simulink model "model_PD"  (R2016b)
settings: Solver=VariableStepAuto  StartTime=0.0  StopTime=30  FixedStep=Ts  RelTol=1e-3  EnableMultiTasking=on
values from neighbouring files (symbols this model uses):
  C = [eye(3),zeros(3,9);zeros(3,6),eye(3),zeros(3,3);zeros(3,9),eye(3)]    [model_script_Cascade.m]    (also in model_script_LQR_LQI.m; model_script_PD.m)
  D_height = .6117    (= 0.6117)    [model_script_Cascade.m]    (also in model_script_PD.m)
  D_pitch = .2256    (= 0.2256)    [model_script_Cascade.m]    (also in model_script_PD.m)
  D_roll = 0.1522    [model_script_Cascade.m]    (also in model_script_PD.m)
  D_yaw = .0367    (= 0.0367)    [model_script_Cascade.m]    (also in model_script_PD.m)
  g = 9.81    [model_script_Cascade.m]    (also in model_script_LQR_LQI.m; model_script_PD.m)
  I = diag([Ixx;Iyy;Izz])    [model_script_Cascade.m]    (also in model_script_LQR_LQI.m; model_script_PD.m)
  i0 = [tauphi;tautheta;taupsi;T]    [model_script_Cascade.m]    (also in model_script_LQR_LQI.m; model_script_PD.m)
  M = 0.487    [model_script_Cascade.m]    (also in model_script_LQR_LQI.m; model_script_PD.m)
  mean_att = zeros(3,1)    [model_script_Cascade.m]    (also in model_script_LQR_LQI.m; model_script_PD.m)
  mean_av = zeros(3,1)    [model_script_Cascade.m]    (also in model_script_LQR_LQI.m; model_script_PD.m)
  mean_pos = zeros(3,1)    [model_script_Cascade.m]    (also in model_script_LQR_LQI.m; model_script_PD.m)
  P_height = .3843    (= 0.3843)    [model_script_Cascade.m]    (also in model_script_PD.m)
  P_pitch = 1.9491    [model_script_Cascade.m]    (also in model_script_PD.m)
  P_roll = 1.5117    [model_script_Cascade.m]    (also in model_script_PD.m)
  P_yaw = .1152    (= 0.1152)    [model_script_Cascade.m]    (also in model_script_PD.m)
  propDistance = 0.125    [model_script_Cascade.m]    (also in model_script_LQR_LQI.m; model_script_PD.m)
  Q = diag([1e-5,1e-5,1e-5,1e-7,1e-7,1e-4,ones(1,2)*2e-7,6e-7,ones(1,3)*1e-7])    [model_script_Cascade.m]    (also in model_script_LQR_LQI.m; model_script_PD.m)
  R = diag(var)    [model_script_Cascade.m]    (also in model_script_LQR_LQI.m; model_script_PD.m)
  T_att = 1/200    (= 0.005)    [model_script_Cascade.m]    (also in model_script_LQR_LQI.m; model_script_PD.m)
  T_xy = 1/10    (= 0.1)    [model_script_Cascade.m]    (also in model_script_LQR_LQI.m; model_script_PD.m)
  T_yaw = 1/100    (= 0.01)    [model_script_Cascade.m]    (also in model_script_LQR_LQI.m; model_script_PD.m)
  T_z = 1/25    (= 0.04)    [model_script_Cascade.m]    (also in model_script_LQR_LQI.m; model_script_PD.m)
  var_att = [9.44454290406988e-06 1.41319492944844e-05 0.000590278082576831]'    [model_script_Cascade.m]    (also in model_script_LQR_LQI.m; model_script_PD.m)
  var_av = [8.38442613623844e-07 9.65548247114005e-07 1.06378940883219e-06]'    [model_script_Cascade.m]    (also in model_script_LQR_LQI.m; model_script_PD.m)
  var_pos = ones(3,1)*0.00219628793119666    [model_script_Cascade.m]    (also in model_script_LQR_LQI.m; model_script_PD.m)
  xi0 = [x;y;z;u;v;w;phi;theta;psi;p;q;r]    [model_script_Cascade.m]    (also in model_script_LQR_LQI.m; model_script_PD.m)
  yawTorqueC = 5    [model_script_Cascade.m]    (also in model_script_LQR_LQI.m; model_script_PD.m)
undefined symbols (not defined in the file or in its folder): den_phi_d, den_theta_d, den_z_d, num_phi_d, num_theta_d, num_z_d, sigbuilder_block, T_pos
undefined symbols (not defined in the file): dronePowerScaling
libraries: aerolibutil x2, simulink x2
(part 2 of 2)

== matlab function model_PD/EKF/Extended Kalman Filter ==
  data: m input; xi input; i input; P_post_prev input; xi_post output; C input; Q input; R input; P_post output; c input; c output
function [xi_post,P_post,c] = fcn(m,xi,i,P_post_prev,C,Q,R,c)
%% Prediction
x = xi(1);      y     = xi(2);      z   = xi(3);
u = xi(4);      v     = xi(5);      w   = xi(6);
phi = xi(7);    theta = xi(8);      psi = xi(9);
p   = xi(10);   q     = xi(11);     r   = xi(12);

tauphi = i(1);  tautheta = i(2);
taupsi = i(3);  T = i(4);

xi_prio = ...
[x - (v*(cos(conj(phi))*sin(conj(psi)) - cos(conj(psi))*sin(conj(phi))*sin(conj(theta))))/400 + (w*(sin(conj(phi))*sin(conj(psi)) + cos(conj(phi))*cos(conj(psi))*sin(conj(theta))))/400 + (u*cos(conj(psi))*cos(conj(theta)))/400;
 y + (v*(cos(conj(phi))*cos(conj(psi)) + sin(conj(phi))*sin(conj(psi))*sin(conj(theta))))/400 - (w*(cos(conj(psi))*sin(conj(phi)) - cos(conj(phi))*sin(conj(psi))*sin(conj(theta))))/400 + (u*cos(conj(theta))*sin(conj(psi)))/400;
                                                                                                                  z - (u*sin(conj(theta)))/400 + (w*cos(conj(phi))*cos(conj(theta)))/400 + (v*cos(conj(theta))*sin(conj(phi)))/400;
                                                                                                                                                                                u - (981*sin(theta))/40000 - (q*w)/400 + (r*v)/400;
                                                                                                                                                                       v + (981*cos(theta)*sin(phi))/40000 + (p*w)/400 - (r*u)/400;
                                                                                                                                                           w - (5*T)/974 + (981*cos(phi)*cos(theta))/40000 - (p*v)/400 + (q*u)/400;
                                                                                                                                                           p/400 + phi + (r*cos(phi)*tan(theta))/400 + (q*sin(phi)*tan(theta))/400;
                                                                                                                                                                                       theta + (q*cos(phi))/400 - (r*sin(phi))/400;
                                                                                                                                                               psi + (r*cos(phi))/(400*cos(theta)) + (q*sin(phi))/(400*cos(theta));
                                                                                                                                                                                                  p + (5*tauphi)/4 - (43*q*r)/8000;
                                                                                                                                                                                              q + (25*tautheta)/16 + (39*p*r)/6400;
                                                                                                                                                                                                   r + (25*taupsi)/59 + (p*q)/5900];

A = ...
[1, 0, 0, (cos(conj(psi))*cos(conj(theta)))/400, (cos(conj(psi))*sin(conj(phi))*sin(conj(theta)))/400 - (cos(conj(phi))*sin(conj(psi)))/400, (sin(conj(phi))*sin(conj(psi)))/400 + (cos(conj(phi))*cos(conj(psi))*sin(conj(theta)))/400,   (v*(sin(conj(phi))*sin(conj(psi)) + cos(conj(phi))*cos(conj(psi))*sin(conj(theta))))/400 + (w*(cos(conj(phi))*sin(conj(psi)) - cos(conj(psi))*sin(conj(phi))*sin(conj(theta))))/400, (w*cos(conj(phi))*cos(conj(psi))*cos(conj(theta)))/400 - (u*cos(conj(psi))*sin(conj(theta)))/400 + (v*cos(conj(psi))*cos(conj(theta))*sin(conj(phi)))/400, (w*(cos(conj(psi))*sin(conj(phi)) - cos(conj(phi))*sin(conj(psi))*sin(conj(theta))))/400 - (v*(cos(conj(phi))*cos(conj(psi)) + sin(conj(phi))*sin(conj(psi))*sin(conj(theta))))/400 - (u*cos(conj(theta))*sin(conj(psi)))/400,           0,                         0,                         0;
 0, 1, 0, (cos(conj(theta))*sin(conj(psi)))/400, (cos(conj(phi))*cos(conj(psi)))/400 + (sin(conj(phi))*sin(conj(psi))*sin(conj(theta)))/400, (cos(conj(phi))*sin(conj(psi))*sin(conj(theta)))/400 - (cos(conj(psi))*sin(conj(phi)))/400, - (v*(cos(conj(psi))*sin(conj(phi)) - cos(conj(phi))*sin(conj(psi))*sin(conj(theta))))/400 - (w*(cos(conj(phi))*cos(conj(psi)) + sin(conj(phi))*sin(conj(psi))*sin(conj(theta))))/400, (w*cos(conj(phi))*cos(conj(theta))*sin(conj(psi)))/400 - (u*sin(conj(psi))*sin(conj(theta)))/400 + (v*cos(conj(theta))*sin(conj(phi))*sin(conj(psi)))/400, (w*(sin(conj(phi))*sin(conj(psi)) + cos(conj(phi))*cos(conj(psi))*sin(conj(theta))))/400 - (v*(cos(conj(phi))*sin(conj(psi)) - cos(conj(psi))*sin(conj(phi))*sin(conj(theta))))/400 + (u*cos(conj(psi))*cos(conj(theta)))/400,           0,                         0,                         0;
 0, 0, 1,                 -sin(conj(theta))/400,                                                      (cos(conj(theta))*sin(conj(phi)))/400,                                                      (cos(conj(phi))*cos(conj(theta)))/400,                                                                                                     (v*cos(conj(phi))*cos(conj(theta)))/400 - (w*cos(conj(theta))*sin(conj(phi)))/400,                                            - (u*cos(conj(theta)))/400 - (w*cos(conj(phi))*sin(conj(theta)))/400 - (v*sin(conj(phi))*sin(conj(theta)))/400,                                                                                                                                                                                                                             0,           0,                         0,                         0;
 0, 0, 0,                                     1,                                                                                      r/400,                                                                                     -q/400,                                                                                                                                                                                     0,                                                                                                                                   -(981*cos(theta))/40000,                                                                                                                                                                                                                             0,           0,                    -w/400,                     v/400;
 0, 0, 0,                                -r/400,                                                                                          1,                                                                                      p/400,                                                                                                                                                       (981*cos(phi)*cos(theta))/40000,                                                                                                                          -(981*sin(phi)*sin(theta))/40000,                                                                                                                                                                                                                             0,       w/400,                         0,                    -u/400;
 0, 0, 0,                                 q/400,                                                                                     -p/400,                                                                                          1,                                                                                                                                                      -(981*cos(theta)*sin(phi))/40000,                                                                                                                          -(981*cos(phi)*sin(theta))/40000,                                                                                                                                                                                                                             0,      -v/400,                     u/400,                         0;
 0, 0, 0,                                     0,                                                                                          0,                                                                                          0,                                                                                                                         (q*cos(phi)*tan(theta))/400 - (r*sin(phi)*tan(theta))/400 + 1,                                                                                 (r*cos(phi)*(tan(theta)^2 + 1))/400 + (q*sin(phi)*(tan(theta)^2 + 1))/400,                                                                                                                                                                                                                             0,       1/400, (sin(phi)*tan(theta))/400, (cos(phi)*tan(theta))/400;
 0, 0, 0,                                     0,                                                                                          0,                                                                                          0,                                                                                                                                                 - (r*cos(phi))/400 - (q*sin(phi))/400,                                                                                                                                                         1,                                                                                                                                                                                                                             0,           0,              cos(phi)/400,             -sin(phi)/400;
 0, 0, 0,                                     0,                                                                                          0,                                                                                          0,                                                                                                                         (q*cos(phi))/(400*cos(theta)) - (r*sin(phi))/(400*cos(theta)),                                                                   (r*cos(phi)*sin(theta))/(400*cos(theta)^2) + (q*sin(phi)*sin(theta))/(400*cos(theta)^2),                                                                                                                                                                                                                             1,           0, sin(phi)/(400*cos(theta)), cos(phi)/(400*cos(theta));
 0, 0, 0,                                     0,                                                                                          0,                                                                                          0,                                                                                                                                                                                     0,                                                                                                                                                         0,                                                                                                                                                                                                                             0,           1,              -(43*r)/8000,              -(43*q)/8000;
 0, 0, 0,                                     0,                                                                                          0,                                                                                          0,                                                                                                                                                                                     0,                                                                                                                                                         0,                                                                                                                                                                                                                             0, (39*r)/6400,                         1,               (39*p)/6400;
 0, 0, 0,                                     0,                                                                                          0,                                                                                          0,                                                                                                                                                                                     0,                                                                                                                                                         0,                                                                                                                                                                                                                             0,      q/5900,                    p/5900,                         1];

P_prio = A*P_post_prev*A'+Q;

%% Update
K = P_prio*C'/(C*P_prio*C'+R);

% Only update states where new sensor data is received
if mod(c,2) ~= 0
    K(:,4:5) = 0;
    K(:,7:9) = 0;
end
if mod(c,4) ~= 0
    K(:,6) = 0;
end
if mod(c,16) ~= 0
    K(:,3) = 0;
end
if mod(c,40) ~= 0
    K(:,1:2) = 0;
end
c = c+1;
if c == 80
    c = 0;
end

% Update states and covariance matrix
xi_post = xi_prio + K*(m-C*xi_prio);
P_post = (eye(size(P_prio,1))-K*C)*P_prio*(eye(size(P_prio,1))-K*C)'+K*R*K';

== matlab function model_PD/Dynamics/Dynamics/Rotation matrices/Rotm in euler ==
  data: alpha input; Rbv output
function Rbv = fcn(alpha)
Rbv = [1,0,0;0,cos(alpha(1)),sin(alpha(1));0,-sin(alpha(1)),cos(alpha(1))]*...
      [cos(alpha(2)),0,-sin(alpha(2));0,1,0;sin(alpha(2)),0,cos(alpha(2))]*...
      [cos(alpha(3)),sin(alpha(3)),0;-sin(alpha(3)),cos(alpha(3)),0;0,0,1];

== matlab function model_PD/Dynamics/Dynamics/equation 7/MATLAB Function ==
  data: alpha input; E output
function E = fcn(alpha)
E = [1, sin(alpha(1))*tan(alpha(2)),cos(alpha(1))*tan(alpha(2));...
     0,               cos(alpha(1)),             -sin(alpha(1));...
     0, sin(alpha(1))/cos(alpha(2)),cos(alpha(1))/cos(alpha(2))];

== matlab function model_PD/Real motor input/Newton To PWM ==
  data: thrustIn input; PWM output; dronePowerScaling parameter
function PWM  = newtonToPWM(thrustIn, dronePowerScaling)

%% Base parameters for PWM to Thrust quadratic fit a*x^2 + b*x + c
% Apply drone power scaling to match the base fit between different drones
a = 0.0001116 * dronePowerScaling;
b = 0.005502 * dronePowerScaling;
c = 0.1036 * dronePowerScaling;

%% Compute desired PWM by inverting the quadratic relationship
d = b * b - 4 * a * (c - thrustIn);
PWM = 0 * thrustIn;
% Ensure no imaginary numbers are computed and PWM doesnt become negative
if d >0 
    candidatePWM = (-b + sqrt(d))/(2 * a);        
    PWM = candidatePWM;
end
